simulink library "dspmisc"  (Simulink 6.0)
settings: Solver=ode45  SolverMode=SingleTasking  StartTime=0.0  StopTime=10.0  RelTol=1e-3
libraries: simulink x2, dspmathops x1, dspmtrx3 x1
settings Model: Creator=mani  LastModifiedBy=mlongfri  ExtModeAutoUpdateStatusClock=off
settings DataIOCC: SignalLoggingName=logsOut
settings OptimizationCC: BooleanDataType=off
settings DebuggingCC: CheckExecutionContextPreStartOutputMsg=on  CheckExecutionContextRuntimeOutputMsg=on  SolverPrmCheckMsg=none
settings HardwareCC: TargetUnknown=on
settings ModelReferenceCC: UpdateModelReferenceTargets=IfOutOfDate
settings GRTTargetCC: LifeSpan=inf
settings SFSimCC: SFSimApplyToAllLibs=on  SFSimBuildMode=Incremental

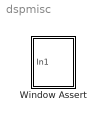
== system dspmisc ==
  Window Assert : Subsystem  EnableExecutionContextPropagation=on  mask{winsize=512, decimat=16, tol=10e-16}
      mask prompts: winsize "Window size:"; decimat "Decimation:"; tol "Tolerance"

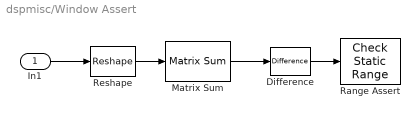
== system dspmisc/Window Assert ==
  In1 : Inport  LatchInput=off
  Difference : dspmathops/Difference  dim=Columns
  Matrix Sum : dspmtrx3/Matrix Sum  Dim=Rows  roundingMode=Floor  overflowMode=off
  Range Assert : simulink/Model Verification/Check  Static Range  Description=-tol <= u <= tol  max=tol  max_included=on  min=-tol  min_included=on  enabled=on  stopWhenAssertionFail=on  export=off  icon=graphic
  Reshape : simulink/Math Operations/Reshape  OutputDimensionality=Customize  OutputDimensions=[decimat, winsize/decimat]
  wires:
  In1/1 -> Reshape/1
  Reshape/1 -> Matrix Sum/1
  Matrix Sum/1 -> Difference/1
  Difference/1 -> Range Assert/1
